simulink model "drone_v2"  (R2017a)
settings: Solver=FixedStepAuto  StartTime=0.0  StopTime=30  FixedStep=0.01  RelTol=1e-3
libraries: simulink x3
settings Model: Creator=mrais  LastModifiedBy=mrais
settings SolverCC: AlgebraicLoopSolver=LineSearch

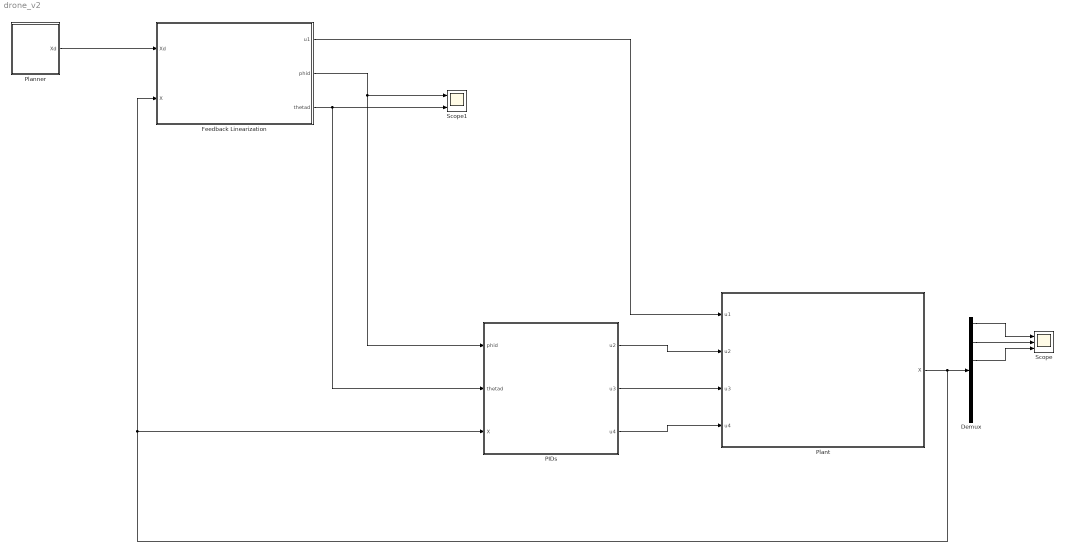
== system drone_v2 ==
  Demux : Demux  Outputs=6
  Feedback Linearization : Subsystem
  PIDs : Subsystem
  Planner : Subsystem
  Plant : Subsystem
  Scope : Scope  NumInputPorts=3
  Scope1 : Scope  NumInputPorts=3
  wires:
  Plant/1(X) -> Feedback Linearization/2(X), PIDs/3(X), Demux/1
  Planner/1(Xd) -> Feedback Linearization/1(Xd)
  Feedback Linearization/1(u1) -> Plant/1(u1)
  Feedback Linearization/2(phid) -> Scope1/1, PIDs/1(phid)
  Feedback Linearization/3(thetad) -> PIDs/2(thetad), Scope1/3
  Demux/3 -> Scope/3
  Demux/1 -> Scope/1
  PIDs/1(u2) -> Plant/2(u2)
  Demux/2 -> Scope/2
  PIDs/2(u3) -> Plant/3(u3)
  PIDs/3(u4) -> Plant/4(u4)

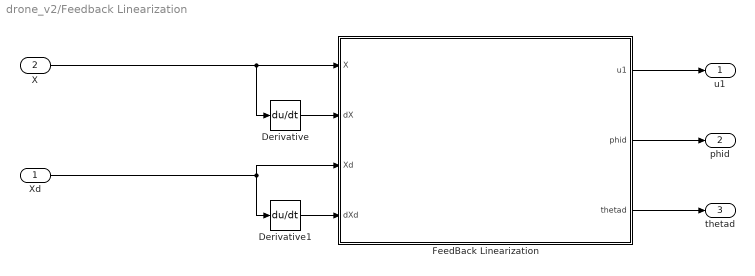
== system drone_v2/Feedback Linearization ==
  Xd : Inport
  X : Inport  Port=2
  Derivative : Derivative
  Derivative1 : Derivative
  FeedBack Linearization : MATLAB Function  TreatAsAtomicUnit=on
  u1 : Outport
  phid : Outport  Port=2
  thetad : Outport  Port=3
  wires:
  Xd/1 -> Derivative1/1, FeedBack Linearization/3(Xd)
  FeedBack Linearization/3(thetad) -> thetad/1
  Derivative/1 -> FeedBack Linearization/2(dX)
  X/1 -> Derivative/1, FeedBack Linearization/1(X)
  FeedBack Linearization/2(phid) -> phid/1
  Derivative1/1 -> FeedBack Linearization/4(dXd)
  FeedBack Linearization/1(u1) -> u1/1

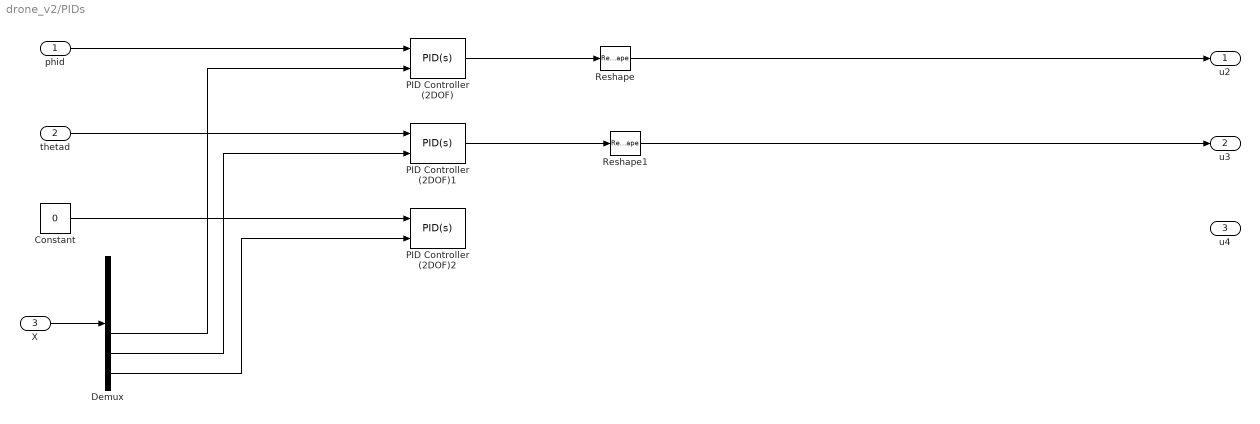
== system drone_v2/PIDs ==
  phid : Inport
  thetad : Inport  Port=2
  X : Inport  Port=3
  Constant : Constant  Value=0
  Demux : Demux  Outputs=6
  PID Controller (2DOF) : simulink/Continuous/PID Controller (2DOF)  Controller=PID  TimeDomain=Continuous-time  SampleTime=-1  IntegratorMethod=Forward Euler  FilterMethod=Forward Euler  Form=Parallel  UseFilter=on  ControllerParametersSource=internal  P=10  I=0  D=10  N=100  b=1  c=1  InitialConditionSource=internal  InitialConditionForIntegrator=0  InitialConditionForFilter=0  ExternalReset=none  LimitOutput=off  UpperSaturationLimit=inf  LowerSaturationLimit=-inf  LinearizeAsGain=on  AntiWindupMode=none  Kb=1  TrackingMode=off  Kt=1  PParamMin=[]  PParamMax=[]  IParamMin=[]  IParamMax=[]  DParamMin=[]  DParamMax=[]  NParamMin=[]  NParamMax=[]  bParamMin=[]  bParamMax=[]  cParamMin=[]  cParamMax=[]  KbParamMin=[]  KbParamMax=[]  KtParamMin=[]  KtParamMax=[]  POutMin=[]  POutMax=[]  IOutMin=[]  IOutMax=[]  DOutMin=[]  DOutMax=[]  NOutMin=[]  NOutMax=[]  bOutMin=[]  bOutMax=[]  cOutMin=[]  cOutMax=[]  KbOutMin=[]  KbOutMax=[]  KtOutMin=[]  KtOutMax=[]  IntegratorOutMin=[]  IntegratorOutMax=[]  FilterOutMin=[]  FilterOutMax=[]  SumOutMin=[]  SumOutMax=[]  Sum1OutMin=[]  Sum1OutMax=[]  Sum2OutMin=[]  Sum2OutMax=[]  Sum3OutMin=[]  Sum3OutMax=[]  SumI1OutMin=[]  SumI1OutMax=[]  SumI2OutMin=[]  SumI2OutMax=[]  SumI3OutMin=[]  SumI3OutMax=[]  SumDOutMin=[]  SumDOutMax=[]  SaturationOutMin=[]  SaturationOutMax=[]  IntegratorContinuousStateAttributes=''  IntegratorStateMustResolveToSignalObject=off  IntegratorRTWStateStorageClass=Auto  FilterContinuousStateAttributes=''  FilterStateMustResolveToSignalObject=off  FilterRTWStateStorageClass=Auto  DifferentiatorICPrevScaledInput=0  DifferentiatorOutMin=[]  DifferentiatorOutMax=[]  InitialConditionSetting=State (most efficient)
  PID Controller (2DOF)1 : simulink/Continuous/PID Controller (2DOF)  Controller=PID  TimeDomain=Continuous-time  SampleTime=-1  IntegratorMethod=Forward Euler  FilterMethod=Forward Euler  Form=Parallel  UseFilter=on  ControllerParametersSource=internal  P=10  I=0  D=10  N=100  b=1  c=1  InitialConditionSource=internal  InitialConditionForIntegrator=0  InitialConditionForFilter=0  ExternalReset=none  LimitOutput=off  UpperSaturationLimit=inf  LowerSaturationLimit=-inf  LinearizeAsGain=on  AntiWindupMode=none  Kb=1  TrackingMode=off  Kt=1  PParamMin=[]  PParamMax=[]  IParamMin=[]  IParamMax=[]  DParamMin=[]  DParamMax=[]  NParamMin=[]  NParamMax=[]  bParamMin=[]  bParamMax=[]  cParamMin=[]  cParamMax=[]  KbParamMin=[]  KbParamMax=[]  KtParamMin=[]  KtParamMax=[]  POutMin=[]  POutMax=[]  IOutMin=[]  IOutMax=[]  DOutMin=[]  DOutMax=[]  NOutMin=[]  NOutMax=[]  bOutMin=[]  bOutMax=[]  cOutMin=[]  cOutMax=[]  KbOutMin=[]  KbOutMax=[]  KtOutMin=[]  KtOutMax=[]  IntegratorOutMin=[]  IntegratorOutMax=[]  FilterOutMin=[]  FilterOutMax=[]  SumOutMin=[]  SumOutMax=[]  Sum1OutMin=[]  Sum1OutMax=[]  Sum2OutMin=[]  Sum2OutMax=[]  Sum3OutMin=[]  Sum3OutMax=[]  SumI1OutMin=[]  SumI1OutMax=[]  SumI2OutMin=[]  SumI2OutMax=[]  SumI3OutMin=[]  SumI3OutMax=[]  SumDOutMin=[]  SumDOutMax=[]  SaturationOutMin=[]  SaturationOutMax=[]  IntegratorContinuousStateAttributes=''  IntegratorStateMustResolveToSignalObject=off  IntegratorRTWStateStorageClass=Auto  FilterContinuousStateAttributes=''  FilterStateMustResolveToSignalObject=off  FilterRTWStateStorageClass=Auto  DifferentiatorICPrevScaledInput=0  DifferentiatorOutMin=[]  DifferentiatorOutMax=[]  InitialConditionSetting=State (most efficient)
  PID Controller (2DOF)2 : simulink/Continuous/PID Controller (2DOF)  Controller=PID  TimeDomain=Continuous-time  SampleTime=-1  IntegratorMethod=Forward Euler  FilterMethod=Forward Euler  Form=Parallel  UseFilter=on  ControllerParametersSource=internal  P=10  I=10  D=10  N=100  b=1  c=1  InitialConditionSource=internal  InitialConditionForIntegrator=0  InitialConditionForFilter=0  ExternalReset=none  LimitOutput=off  UpperSaturationLimit=inf  LowerSaturationLimit=-inf  LinearizeAsGain=on  AntiWindupMode=none  Kb=1  TrackingMode=off  Kt=1  PParamMin=[]  PParamMax=[]  IParamMin=[]  IParamMax=[]  DParamMin=[]  DParamMax=[]  NParamMin=[]  NParamMax=[]  bParamMin=[]  bParamMax=[]  cParamMin=[]  cParamMax=[]  KbParamMin=[]  KbParamMax=[]  KtParamMin=[]  KtParamMax=[]  POutMin=[]  POutMax=[]  IOutMin=[]  IOutMax=[]  DOutMin=[]  DOutMax=[]  NOutMin=[]  NOutMax=[]  bOutMin=[]  bOutMax=[]  cOutMin=[]  cOutMax=[]  KbOutMin=[]  KbOutMax=[]  KtOutMin=[]  KtOutMax=[]  IntegratorOutMin=[]  IntegratorOutMax=[]  FilterOutMin=[]  FilterOutMax=[]  SumOutMin=[]  SumOutMax=[]  Sum1OutMin=[]  Sum1OutMax=[]  Sum2OutMin=[]  Sum2OutMax=[]  Sum3OutMin=[]  Sum3OutMax=[]  SumI1OutMin=[]  SumI1OutMax=[]  SumI2OutMin=[]  SumI2OutMax=[]  SumI3OutMin=[]  SumI3OutMax=[]  SumDOutMin=[]  SumDOutMax=[]  SaturationOutMin=[]  SaturationOutMax=[]  IntegratorContinuousStateAttributes=''  IntegratorStateMustResolveToSignalObject=off  IntegratorRTWStateStorageClass=Auto  FilterContinuousStateAttributes=''  FilterStateMustResolveToSignalObject=off  FilterRTWStateStorageClass=Auto  DifferentiatorICPrevScaledInput=0  DifferentiatorOutMin=[]  DifferentiatorOutMax=[]  InitialConditionSetting=State (most efficient)
  Reshape : Reshape  OutputDimensionality=Customize
  Reshape1 : Reshape  OutputDimensionality=Customize
  u2 : Outport
  u3 : Outport  Port=2
  u4 : Outport  Port=3
  wires:
  PID Controller (2DOF)/1 -> Reshape/1
  thetad/1 -> PID Controller (2DOF)1/1
  phid/1 -> PID Controller (2DOF)/1
  PID Controller (2DOF)1/1 -> Reshape1/1
  Constant/1 -> PID Controller (2DOF)2/1
  X/1 -> Demux/1
  Demux/4 -> PID Controller (2DOF)/2
  Demux/5 -> PID Controller (2DOF)1/2
  Demux/6 -> PID Controller (2DOF)2/2
  Reshape1/1 -> u3/1
  Reshape/1 -> u2/1

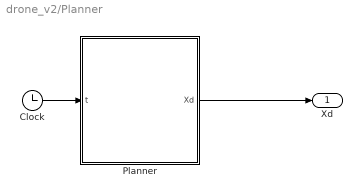
== system drone_v2/Planner ==
  Clock : Clock
  Planner : MATLAB Function  TreatAsAtomicUnit=on
  Xd : Outport
  wires:
  Clock/1 -> Planner/1(t)
  Planner/1(Xd) -> Xd/1

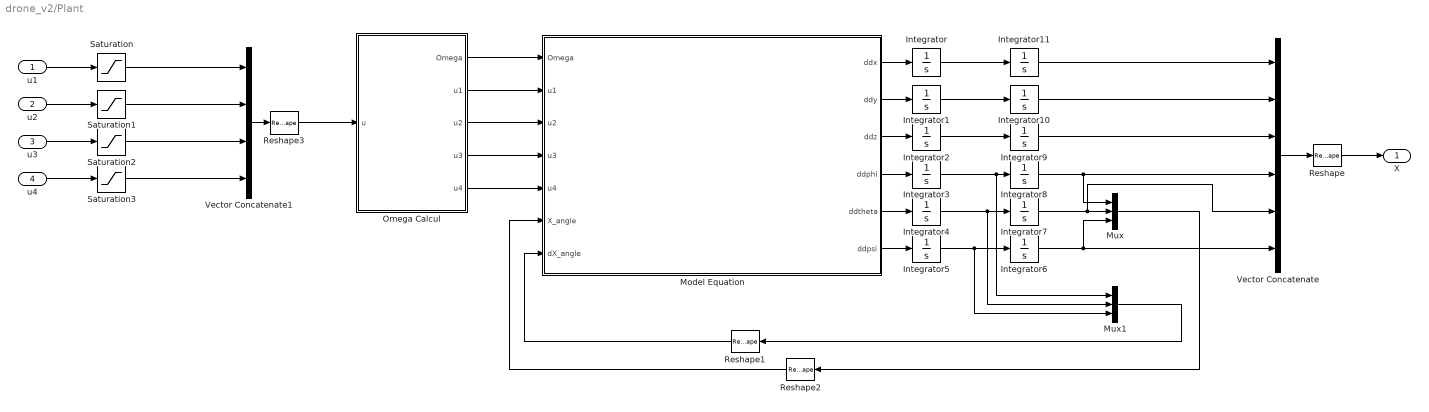
== system drone_v2/Plant ==
  u1 : Inport
  u2 : Inport  Port=2
  u3 : Inport  Port=3
  u4 : Inport  Port=4
  Integrator{,1..11} (12 alike) : Integrator
  Model Equation : MATLAB Function  TreatAsAtomicUnit=on
  Mux : Mux  Inputs=3
  Mux1 : Mux  Inputs=3
  Omega Calcul : MATLAB Function  TreatAsAtomicUnit=on
  Reshape : Reshape  OutputDimensionality=Customize  OutputDimensions=[1,6]
  Reshape1 : Reshape  OutputDimensionality=Customize  OutputDimensions=[1,3]
  Reshape2 : Reshape  OutputDimensionality=Customize  OutputDimensions=[1,3]
  Reshape3 : Reshape  OutputDimensionality=Customize  OutputDimensions=[4,1]
  Saturation : Saturate  UpperLimit=65  LowerLimit=0
  Saturation1 : Saturate  UpperLimit=2.85  LowerLimit=-2.85
  Saturation2 : Saturate  UpperLimit=2.85  LowerLimit=-2.85
  Saturation3 : Saturate  UpperLimit=1.17  LowerLimit=-1.17
  Vector Concatenate : Concatenate  NumInputs=6  Mode=Multidimensional array  ConcatenateDimension=2
  Vector Concatenate1 : Concatenate  NumInputs=4  Mode=Multidimensional array
  X : Outport
  wires:
  Model Equation/5(ddtheta) -> Integrator4/1
  Integrator5/1 -> Mux1/3, Integrator6/1
  Integrator8/1 -> Vector Concatenate/4, Mux/1
  Integrator3/1 -> Mux1/1, Integrator8/1
  Integrator/1 -> Integrator11/1
  Integrator4/1 -> Mux1/2, Integrator7/1
  Mux1/1 -> Reshape1/1
  Model Equation/3(ddz) -> Integrator2/1
  Model Equation/1(ddx) -> Integrator/1
  Integrator6/1 -> Vector Concatenate/6, Mux/3
  Integrator7/1 -> Vector Concatenate/5, Mux/2
  Mux/1 -> Reshape2/1
  Integrator2/1 -> Integrator9/1
  Vector Concatenate/1 -> Reshape/1
  Model Equation/4(ddphi) -> Integrator3/1
  Integrator1/1 -> Integrator10/1
  Model Equation/6(ddpsi) -> Integrator5/1
  Integrator11/1 -> Vector Concatenate/1
  Integrator10/1 -> Vector Concatenate/2
  Model Equation/2(ddy) -> Integrator1/1
  Integrator9/1 -> Vector Concatenate/3
  Reshape/1 -> X/1
  Reshape2/1 -> Model Equation/6(X_angle)
  Reshape1/1 -> Model Equation/7(dX_angle)
  Vector Concatenate1/1 -> Reshape3/1
  u1/1 -> Saturation/1
  u2/1 -> Saturation1/1
  u3/1 -> Saturation2/1
  u4/1 -> Saturation3/1
  Reshape3/1 -> Omega Calcul/1(u)
  Omega Calcul/1(Omega) -> Model Equation/1(Omega)
  Saturation/1 -> Vector Concatenate1/1
  Saturation1/1 -> Vector Concatenate1/2
  Saturation2/1 -> Vector Concatenate1/3
  Saturation3/1 -> Vector Concatenate1/4
  Omega Calcul/2(u1) -> Model Equation/2(u1)
  Omega Calcul/3(u2) -> Model Equation/3(u2)
  Omega Calcul/4(u3) -> Model Equation/4(u3)
  Omega Calcul/5(u4) -> Model Equation/5(u4)

== matlab function drone_v2/Plant/Model Equation ==
  data: Omega input; ddx output; u1 input; u2 input; u3 input; u4 input; X_angle input; dX_angle input; ddy output; ddz output; ddphi output; ddtheta output; ddpsi output
function [ddx, ddy, ddz, ddphi, ddtheta, ddpsi] = fcn(Omega, u1, u2, u3, u4, X_angle, dX_angle)

constant = initial_constants();
Ix = constant{1}; Iy = constant{2}; Iz = constant{3}; 
m = constant{4};
g = constant{5};
Jr = constant{6};
l = constant{9};

phi = X_angle(1); theta = X_angle(2); psi = X_angle(3);
dphi = dX_angle(1); dtheta = dX_angle(2); dpsi = dX_angle(3);


ddx = (cos(phi)*sin(theta)*cos(psi) + sin(phi)*sin(psi))*u1/m;
ddy = (cos(phi)*sin(theta)*sin(psi) - sin(phi)*cos(psi))*u1/m;
ddz = -g + cos(phi)*cos(theta)*u1/m;

ddphi = dphi*dpsi*((Iy - Iz)/Ix) - Jr*dtheta*Omega/Ix + l*u2/Ix;
ddtheta = dphi*dpsi*((Iz - Ix)/Iy) + Jr*dtheta*Omega/Iy + l*u3/Iy;
ddpsi = dtheta*dphi*((Ix - Iy)/Iz) + u4/Iz;

== matlab function drone_v2/Planner/Planner ==
  data: Xd output; t input
function Xd  = fcn(t)

R=10;
zt = 0;
xt = (R+2)*sin(t/2);
yt = 0;
Xd = [xt, yt, zt];

end

== matlab function drone_v2/Feedback Linearization/FeedBack Linearization ==
  data: X input; dX input; Xd input; dXd input; u1 output; phid output; thetad output
function [u1, phid, thetad] = fcn(X, dX, Xd, dXd)
constant = initial_constants();
g = constant{5};
m = constant{4};

k1x = 1; k2x = 2;
k1y = 1; k2y =2;
k1z = 1; k2z =2;

x = X(1); y = X(2); z = X(3); phi = X(4); theta = X(5); psi = X(6);
dx = dX(1); dy = dX(2); dz = dX(3);
xd = Xd(1); yd = Xd(2); zd = Xd(3); 
dxd = dXd(1); dyd = dXd(2); dzd = dXd(3); 



vx = k1x*(xd - x) + k2x*(dxd - dx);
vy = k1y*(yd - y) + k2y*(dyd - dy);
vz = k1z*(zd - z) + k2z*(dzd - dz);

a = vx /(vz + g); 
b = vy /(vz + g); 
c = cos(psi);
d = sin(psi);

u1 = (vz + g)*m/(cos(phi)*cos(theta));
thetad = atan(a*c+b*d);

if abs(psi) < pi/4 || abs(psi) > 3*pi/4
    phid = atan( (cos(theta)*(tan(theta)*d - b))/c);
else
    phid = atan( (cos(theta)*(a - tan(theta)*c))/d);
end



end

== matlab function drone_v2/Plant/Omega Calcul ==
  data: u input; Omega output; u1 output; u2 output; u3 output; u4 output
function [Omega, u1, u2, u3, u4] = fcn(u)

constant = initial_constants();
cT = constant{7};
cQ = constant{8};
l  = constant{9};
u1C = u(1)/cT;
u2C = u(2)/(cT*l);
u3C = u(3)/(cT*l);
u4C = u(4)/cQ;

omega4P2 = (u1C + 2*u2C + u4C)/4;
omega3P2 = (-u4C + 2*omega4P2 - u2C + u3C)/2;
omega2P2 = omega4P2 - u2C;
omega1P2 = omega3P2 - u3C;

Omegas_square = [omega1P2, omega2P2, omega3P2, omega4P2]
Omegas = sqrt(abs(Omegas_square));
Omegas(Omegas > 14800) = 14800; % max vitesse rotation d'un moteur 1000 kV alimenté par lipo 4S

Omega = -Omegas(1) + Omegas(2) - Omegas(3) + Omegas(4);
u_aux = [cT*(Omegas(1)^2 + Omegas(2)^2 + Omegas(3)^2 + Omegas(4)^2),
         cT*l*(Omegas(4)^2 - Omegas(2)^2),
         cT*l*(Omegas(3)^2 - Omegas(1)^2),
         cQ*(-Omegas(1)^2 + Omegas(2)^2 - Omegas(3)^2 + Omegas(4)^2)];

u1 = u_aux(1)
u2 = u_aux(2)
u3 = u_aux(3)
u4 = u_aux(4)

end
